simulink model "ServoControl"  (R2014a)
settings: Solver=ode45  StartTime=0.0  StopTime=10.0  RelTol=1e-3
libraries: hdlsllib x2, simulink x1
settings Model: Creator=amir  LastModifiedBy=massucco.j
settings OptimizationCC: BlockReduction=off  ConditionallyExecuteInputs=off  InlineParams=on
settings DebuggingCC: AlgebraicLoopMsg=error  MergeDetectMultiDrivingBlocksExec=error
settings HardwareCC: ProdHWDeviceType=ASIC/FPGA->ASIC/FPGA  ProdEqTarget=off

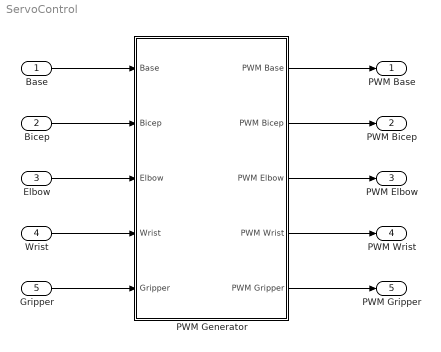
== system ServoControl ==
  Base : Inport  OutDataTypeStr=uint8  SampleTime=1
  Bicep : Inport  Port=2  OutDataTypeStr=uint8  SampleTime=1
  Elbow : Inport  Port=3  OutDataTypeStr=uint8  SampleTime=1
  Wrist : Inport  Port=4  OutDataTypeStr=uint8  SampleTime=1
  Gripper : Inport  Port=5  OutDataTypeStr=uint8  SampleTime=1
  PWM Generator : Subsystem  TreatAsAtomicUnit=on
  PWM Base : Outport
  PWM Bicep : Outport  Port=2
  PWM Elbow : Outport  Port=3
  PWM Wrist : Outport  Port=4
  PWM Gripper : Outport  Port=5
  wires:
  Base/1 -> PWM Generator/1(Base)
  Bicep/1 -> PWM Generator/2(Bicep)
  Elbow/1 -> PWM Generator/3(Elbow)
  Wrist/1 -> PWM Generator/4(Wrist)
  Gripper/1 -> PWM Generator/5(Gripper)
  PWM Generator/1(PWM Base) -> PWM Base/1
  PWM Generator/2(PWM Bicep) -> PWM Bicep/1
  PWM Generator/3(PWM Elbow) -> PWM Elbow/1
  PWM Generator/4(PWM Wrist) -> PWM Wrist/1
  PWM Generator/5(PWM Gripper) -> PWM Gripper/1

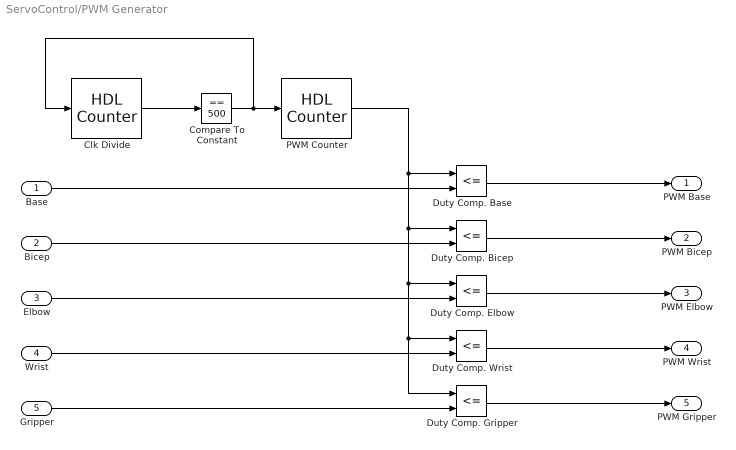
== system ServoControl/PWM Generator ==
  Base : Inport  OutDataTypeStr=uint8  SampleTime=1
  Bicep : Inport  Port=2  OutDataTypeStr=uint8  SampleTime=1
  Elbow : Inport  Port=3  OutDataTypeStr=uint8  SampleTime=1
  Wrist : Inport  Port=4  OutDataTypeStr=uint8  SampleTime=1
  Gripper : Inport  Port=5  OutDataTypeStr=uint8  SampleTime=1
  Clk Divide : hdlsllib/HDL Operations/HDL Counter  CountType=Free running  CountInit=1  CountStep=1  CountMax=500  CountFromType=Initial value  CountFrom=1  CountResetPort=on  CountLoadPort=off  CountEnbPort=off  CountDirPort=off  CountDataType=Unsigned  CountWordLen=16  CountFracLen=0  CountSampTime=1
  Compare To Constant : simulink/Logic and Bit Operations/Compare To Constant  relop===  const=500  OutDataTypeStr=boolean
  Duty Comp. Base : RelationalOperator  Operator=<=  OutDataTypeStr=boolean
  Duty Comp. Bicep : RelationalOperator  Operator=<=  OutDataTypeStr=boolean
  Duty Comp. Elbow : RelationalOperator  Operator=<=  OutDataTypeStr=boolean
  Duty Comp. Gripper : RelationalOperator  Operator=<=  OutDataTypeStr=boolean
  Duty Comp. Wrist : RelationalOperator  Operator=<=  OutDataTypeStr=boolean
  PWM Counter : hdlsllib/HDL Operations/HDL Counter  CountType=Count limited  CountInit=1  CountStep=1  CountMax=2000  CountFromType=Initial value  CountFrom=1  CountResetPort=off  CountLoadPort=off  CountEnbPort=on  CountDirPort=off  CountDataType=Unsigned  CountWordLen=16  CountFracLen=0  CountSampTime=1
  PWM Base : Outport
  PWM Bicep : Outport  Port=2
  PWM Elbow : Outport  Port=3
  PWM Wrist : Outport  Port=4
  PWM Gripper : Outport  Port=5
  wires:
  Clk Divide/1 -> Compare To Constant/1
  Compare To Constant/1 -> Clk Divide/1, PWM Counter/1
  Gripper/1 -> Duty Comp. Gripper/2
  Elbow/1 -> Duty Comp. Elbow/2
  Wrist/1 -> Duty Comp. Wrist/2
  Duty Comp. Elbow/1 -> PWM Elbow/1
  Base/1 -> Duty Comp. Base/2
  PWM Counter/1 -> Duty Comp. Base/1, Duty Comp. Bicep/1, Duty Comp. Elbow/1, Duty Comp. Wrist/1, Duty Comp. Gripper/1
  Bicep/1 -> Duty Comp. Bicep/2
  Duty Comp. Bicep/1 -> PWM Bicep/1
  Duty Comp. Wrist/1 -> PWM Wrist/1
  Duty Comp. Gripper/1 -> PWM Gripper/1
  Duty Comp. Base/1 -> PWM Base/1
